simulink library "RABBIT_lib"  (R2015a)
settings: Solver=ode45  StartTime=0.0  StopTime=10.0  RelTol=1e-3
undefined symbols (not defined in the file or in its folder): dt, RABBITparams
undefined symbols (not defined in the file): RABBITsignals
settings Model: Creator=ffelici  LastModifiedBy=ffelici
settings SFSimCC: SimParseCustomCode=off

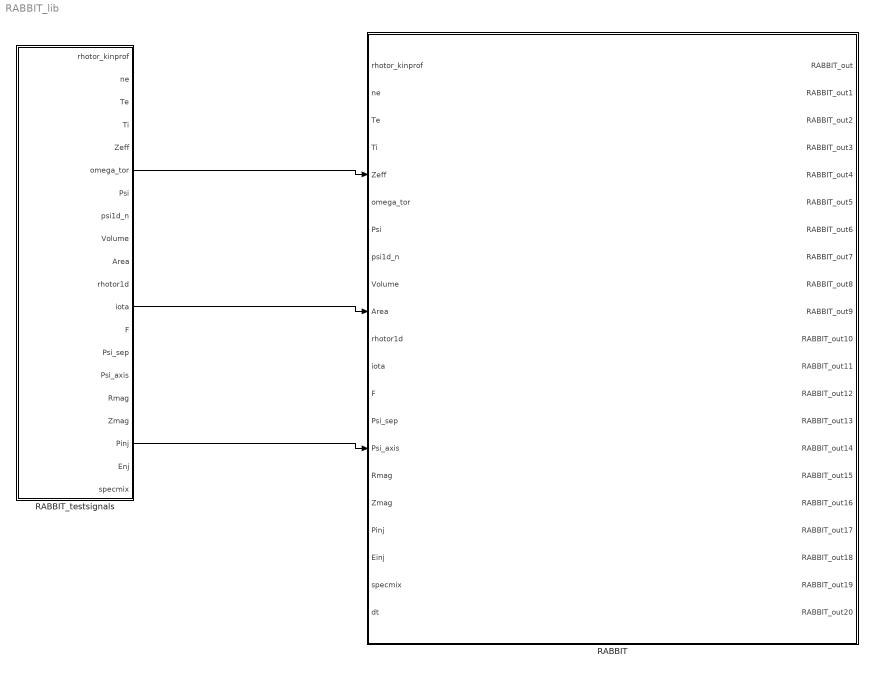
== system RABBIT_lib ==
  RABBIT : Subsystem  mask{RABBITparams=RABBITparams}
      mask prompts: RABBITparams "RABBIT parameters"
      mask Display:
      | image('rabbit.jpg')
      | 
      | port_label('input',1,'rhotorN kin profiles')
      | port_label('input',2,'ne [m^-3]')
      | port_label('input',3,'Te [eV]')
      | port_label('input',4,'Ti [eV]')
      | port_label('input',5,'Zeff')
      | port_label('input',6,'omega tor [rad/s]')
      | port_label('input',7,'Psi 2D [Wb/rad]')
      | port_label('input',8,'Psi1D grid [0-1]')
      | port_label('input',9,'Volume m^3')
      | port_label('input',10,'Area m^2')
      | port_label('input',11,'rhotorN eq profiles')
      | port_label('input',12,'iota = 1/q')
      | port_label('input',13,'F [Tm]')
      | port_label('input',14,'Psi_sep [Wb/rad]')
      | port_label('input',15,'Psi_axis [Wb/rad]')
      | port_label('input',16,'Rmag [m]')
      | port_label('input',17,'Zmag [m]')
      | port_label('input',18,'Pinj [W]')
      | port_label('input',19,'Einj [W]')
      | port_label('input',20,'specmix [-]')
      | port_label('input',21,'dt [s]')
      | 
      | 
      | port_label('output',1,'Power e- [W/m^3]')
      | port_label('output',2,'Power i+ [W/m^3]')
      | port_label('output',3,'Fast ion pressure [Pa]')
      | port_label('output',4,'Particle source [1/m^3/s]')
      | port_label('output',5,'Fast ion density [1/m^3]')
      | port_label('output',6,'Fast ion current density [A/m^2]')
      | port_label('output',7,'NB driven current [A/m^2]')
      | port_label('output',8,'Torque to electrons [Nm/m^3]')
      | port_label('output',9,'Torque to ions [Nm/m^3]')
      | port_label('output',10,'Torque to impurities [Nm/m^3]')
      | port_label('output',11,'Neutron rate [#/s/m^3]')
      | port_label('output',12,'rhotor out [-]')
      | port_label('output',13,'P e- total [W]')
      | port_label('output',14,'P i- total [W]')
      | port_label('output',15,'P shinethrough [W]')
      | port_label('output',16,'P rotation [W]')
      | port_label('output',17,'P orbit loss [W]')
      | port_label('output',18,'P CX loss [W]')
      | port_label('output',19,'Inb total [A]')
      | port_label('output',20,'exitflag')
      | port_label('output',21,'execution time [ms]')
  RABBIT_testsignals : Subsystem  mask{RABBITsignals=RABBITsignals, dt=dt}
      mask prompts: RABBITsignals "RABBITsignals structure"; dt "sample time"
  wires:
  RABBIT_testsignals/6(omega_tor) -> RABBIT/5(Zeff)
  RABBIT_testsignals/12(iota) -> RABBIT/10(Area)
  RABBIT_testsignals/18(Pinj) -> RABBIT/15(Psi_axis)

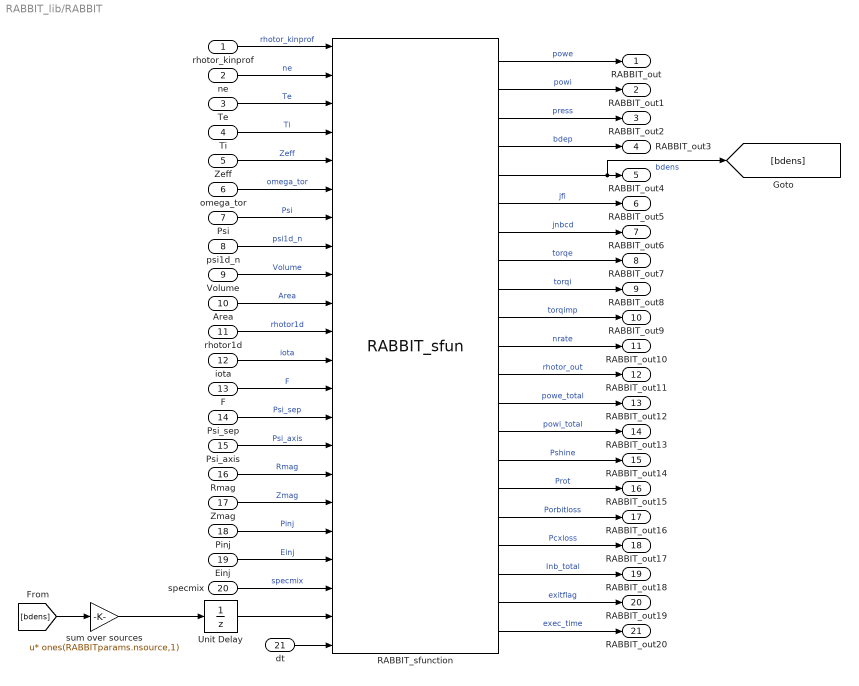
== system RABBIT_lib/RABBIT ==
  rhotor_kinprof : Inport  OutDataTypeStr=double  Interpolate=off
  ne : Inport  Port=2  OutDataTypeStr=double  Interpolate=off
  Te : Inport  Port=3  OutDataTypeStr=double  Interpolate=off
  Ti : Inport  Port=4  OutDataTypeStr=double  Interpolate=off
  Zeff : Inport  Port=5  OutDataTypeStr=double  Interpolate=off
  omega_tor : Inport  Port=6  OutDataTypeStr=double  Interpolate=off
  Psi : Inport  Port=7  OutDataTypeStr=double  Interpolate=off
  psi1d_n : Inport  Port=8  OutDataTypeStr=double  Interpolate=off
  Volume : Inport  Port=9  OutDataTypeStr=double  Interpolate=off
  Area : Inport  Port=10  OutDataTypeStr=double  Interpolate=off
  rhotor1d : Inport  Port=11  OutDataTypeStr=double  Interpolate=off
  iota : Inport  Port=12  OutDataTypeStr=double  Interpolate=off
  F : Inport  Port=13  OutDataTypeStr=double  Interpolate=off
  Psi_sep : Inport  Port=14  OutDataTypeStr=double  Interpolate=off
  Psi_axis : Inport  Port=15  OutDataTypeStr=double  Interpolate=off
  Rmag : Inport  Port=16  OutDataTypeStr=double  Interpolate=off
  Zmag : Inport  Port=17  OutDataTypeStr=double  Interpolate=off
  Pinj : Inport  Port=18  OutDataTypeStr=double  Interpolate=off
  Einj : Inport  Port=19  OutDataTypeStr=double  Interpolate=off
  specmix : Inport  Port=20  OutDataTypeStr=double  Interpolate=off
  dt : Inport  Port=21  OutDataTypeStr=double  PortDimensions=1  Interpolate=off
  RABBIT_sfunction : S-Function  FunctionName=RABBIT_sfun  Parameters=p.nsource,p.aplasma,p.zplasma,p.aimp,p.zimp,p.abeam,p.zbeam,p.xstart,p.xvec,p.beamwidthpoly,p.nv,p.nrhotor_out,p.R,p.Z,p.l,p.p  mask{p=RABBITparams}
      mask prompts: p "RABBITparams structure"
  Unit Delay : UnitDelay  SampleTime=-1
  sum over sources : Gain  Gain=ones(RABBITparams.nsource,1)  Multiplication=Matrix(u*K)
  RABBIT_out : Outport  OutDataTypeStr=double
  RABBIT_out1 : Outport  Port=2  OutDataTypeStr=double
  RABBIT_out2 : Outport  Port=3  OutDataTypeStr=double
  RABBIT_out3 : Outport  Port=4  OutDataTypeStr=double
  RABBIT_out4 : Outport  Port=5  OutDataTypeStr=double
  RABBIT_out5 : Outport  Port=6  OutDataTypeStr=double
  RABBIT_out6 : Outport  Port=7  OutDataTypeStr=double
  RABBIT_out7 : Outport  Port=8  OutDataTypeStr=double
  RABBIT_out8 : Outport  Port=9  OutDataTypeStr=double
  RABBIT_out9 : Outport  Port=10  OutDataTypeStr=double
  RABBIT_out10 : Outport  Port=11  OutDataTypeStr=double
  RABBIT_out11 : Outport  Port=12  OutDataTypeStr=double
  RABBIT_out12 : Outport  Port=13  OutDataTypeStr=double
  RABBIT_out13 : Outport  Port=14  OutDataTypeStr=double
  RABBIT_out14 : Outport  Port=15  OutDataTypeStr=double
  RABBIT_out15 : Outport  Port=16  OutDataTypeStr=double
  RABBIT_out16 : Outport  Port=17  OutDataTypeStr=double
  RABBIT_out17 : Outport  Port=18  OutDataTypeStr=double
  RABBIT_out18 : Outport  Port=19  OutDataTypeStr=double
  RABBIT_out19 : Outport  Port=20  OutDataTypeStr=double
  RABBIT_out20 : Outport  Port=21  OutDataTypeStr=double
  wires:
  Rmag/1 -> RABBIT_sfunction/16  "Rmag"
  RABBIT_sfunction/20 -> RABBIT_out19/1  "exitflag"
  sum over sources/1 -> Unit Delay/1
  dt/1 -> RABBIT_sfunction/22
  Zeff/1 -> RABBIT_sfunction/5  "Zeff"
  psi1d_n/1 -> RABBIT_sfunction/8  "psi1d_n"
  rhotor_kinprof/1 -> RABBIT_sfunction/1  "rhotor_kinprof"
  Te/1 -> RABBIT_sfunction/3  "Te"
  RABBIT_sfunction/14 -> RABBIT_out13/1  "powi_total"
  RABBIT_sfunction/15 -> RABBIT_out14/1  "Pshine"
  RABBIT_sfunction/16 -> RABBIT_out15/1  "Prot"
  RABBIT_sfunction/7 -> RABBIT_out6/1  "jnbcd"
  RABBIT_sfunction/8 -> RABBIT_out7/1  "torqe"
  RABBIT_sfunction/12 -> RABBIT_out11/1  "rhotor_out"
  RABBIT_sfunction/3 -> RABBIT_out2/1  "press"
  RABBIT_sfunction/6 -> RABBIT_out5/1  "jfi"
  RABBIT_sfunction/5 -> [bdens], RABBIT_out4/1  "bdens"
  RABBIT_sfunction/4 -> RABBIT_out3/1  "bdep"
  RABBIT_sfunction/2 -> RABBIT_out1/1  "powi"
  RABBIT_sfunction/1 -> RABBIT_out/1  "powe"
  [bdens] -> sum over sources/1
  Psi_sep/1 -> RABBIT_sfunction/14  "Psi_sep"
  Volume/1 -> RABBIT_sfunction/9  "Volume"
  specmix/1 -> RABBIT_sfunction/20  "specmix"
  Psi/1 -> RABBIT_sfunction/7  "Psi"
  rhotor1d/1 -> RABBIT_sfunction/11  "rhotor1d"
  Einj/1 -> RABBIT_sfunction/19  "Einj"
  Unit Delay/1 -> RABBIT_sfunction/21
  omega_tor/1 -> RABBIT_sfunction/6  "omega_tor"
  ne/1 -> RABBIT_sfunction/2  "ne"
  Ti/1 -> RABBIT_sfunction/4  "Ti"
  Area/1 -> RABBIT_sfunction/10  "Area"
  Psi_axis/1 -> RABBIT_sfunction/15  "Psi_axis"
  RABBIT_sfunction/21 -> RABBIT_out20/1  "exec_time"
  RABBIT_sfunction/19 -> RABBIT_out18/1  "Inb_total"
  RABBIT_sfunction/18 -> RABBIT_out17/1  "Pcxloss"
  RABBIT_sfunction/13 -> RABBIT_out12/1  "powe_total"
  RABBIT_sfunction/17 -> RABBIT_out16/1  "Porbitloss"
  Pinj/1 -> RABBIT_sfunction/18  "Pinj"
  iota/1 -> RABBIT_sfunction/12  "iota"
  F/1 -> RABBIT_sfunction/13  "F"
  RABBIT_sfunction/10 -> RABBIT_out9/1  "torqimp"
  RABBIT_sfunction/9 -> RABBIT_out8/1  "torqi"
  RABBIT_sfunction/11 -> RABBIT_out10/1  "nrate"
  Zmag/1 -> RABBIT_sfunction/17  "Zmag"

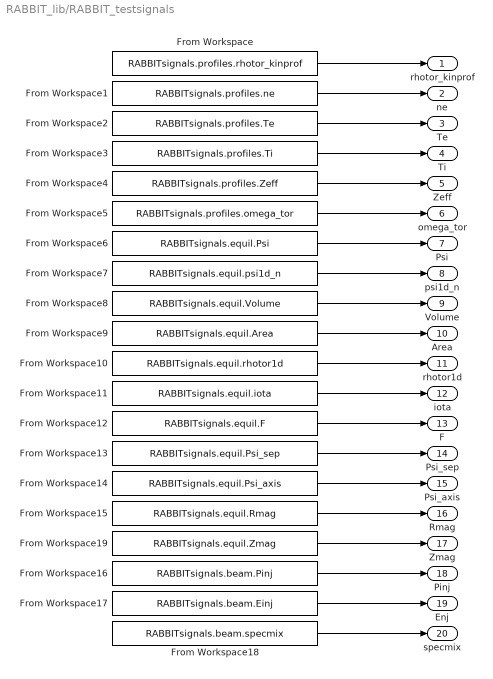
== system RABBIT_lib/RABBIT_testsignals ==
  From Workspace : FromWorkspace  VariableName=RABBITsignals.profiles.rhotor_kinprof  SampleTime=dt  OutputAfterFinalValue=Holding final value
  From Workspace1 : FromWorkspace  VariableName=RABBITsignals.profiles.ne  SampleTime=dt  OutputAfterFinalValue=Holding final value
  From Workspace10 : FromWorkspace  VariableName=RABBITsignals.equil.rhotor1d  SampleTime=dt  OutputAfterFinalValue=Holding final value
  From Workspace11 : FromWorkspace  VariableName=RABBITsignals.equil.iota  SampleTime=dt  OutputAfterFinalValue=Holding final value
  From Workspace12 : FromWorkspace  VariableName=RABBITsignals.equil.F  SampleTime=dt  OutputAfterFinalValue=Holding final value
  From Workspace13 : FromWorkspace  VariableName=RABBITsignals.equil.Psi_sep  SampleTime=dt  OutputAfterFinalValue=Holding final value
  From Workspace14 : FromWorkspace  VariableName=RABBITsignals.equil.Psi_axis  SampleTime=dt  OutputAfterFinalValue=Holding final value
  From Workspace15 : FromWorkspace  VariableName=RABBITsignals.equil.Rmag  SampleTime=dt  OutputAfterFinalValue=Holding final value
  From Workspace16 : FromWorkspace  VariableName=RABBITsignals.beam.Pinj  SampleTime=dt  OutputAfterFinalValue=Holding final value
  From Workspace17 : FromWorkspace  VariableName=RABBITsignals.beam.Einj  SampleTime=dt  OutputAfterFinalValue=Holding final value
  From Workspace18 : FromWorkspace  VariableName=RABBITsignals.beam.specmix  SampleTime=dt  OutputAfterFinalValue=Holding final value
  From Workspace19 : FromWorkspace  VariableName=RABBITsignals.equil.Zmag  SampleTime=dt  OutputAfterFinalValue=Holding final value
  From Workspace2 : FromWorkspace  VariableName=RABBITsignals.profiles.Te  SampleTime=dt  OutputAfterFinalValue=Holding final value
  From Workspace3 : FromWorkspace  VariableName=RABBITsignals.profiles.Ti  SampleTime=dt  OutputAfterFinalValue=Holding final value
  From Workspace4 : FromWorkspace  VariableName=RABBITsignals.profiles.Zeff  SampleTime=dt  OutputAfterFinalValue=Holding final value
  From Workspace5 : FromWorkspace  VariableName=RABBITsignals.profiles.omega_tor  SampleTime=dt  OutputAfterFinalValue=Holding final value
  From Workspace6 : FromWorkspace  VariableName=RABBITsignals.equil.Psi  SampleTime=dt  OutputAfterFinalValue=Holding final value
  From Workspace7 : FromWorkspace  VariableName=RABBITsignals.equil.psi1d_n  SampleTime=dt  OutputAfterFinalValue=Holding final value
  From Workspace8 : FromWorkspace  VariableName=RABBITsignals.equil.Volume  SampleTime=dt  OutputAfterFinalValue=Holding final value
  From Workspace9 : FromWorkspace  VariableName=RABBITsignals.equil.Area  SampleTime=dt  OutputAfterFinalValue=Holding final value
  "  rhotor_kinprof" : Outport
  ne : Outport  Port=2
  Te : Outport  Port=3
  Ti : Outport  Port=4
  Zeff : Outport  Port=5
  omega_tor : Outport  Port=6
  Psi : Outport  Port=7
  psi1d_n : Outport  Port=8
  Volume : Outport  Port=9
  Area : Outport  Port=10
  rhotor1d : Outport  Port=11
  iota : Outport  Port=12
  F : Outport  Port=13
  Psi_sep : Outport  Port=14
  Psi_axis : Outport  Port=15
  Rmag : Outport  Port=16
  Zmag : Outport  Port=17
  Pinj : Outport  Port=18
  Enj : Outport  Port=19
  specmix : Outport  Port=20
  wires:
  From Workspace10/1 -> rhotor1d/1
  From Workspace15/1 -> Rmag/1
  From Workspace13/1 -> Psi_sep/1
  From Workspace11/1 -> iota/1
  From Workspace8/1 -> Volume/1
  From Workspace19/1 -> Zmag/1
  From Workspace9/1 -> Area/1
  From Workspace/1 -> "  rhotor_kinprof"/1
  From Workspace7/1 -> psi1d_n/1
  From Workspace18/1 -> specmix/1
  From Workspace14/1 -> Psi_axis/1
  From Workspace12/1 -> F/1
  From Workspace1/1 -> ne/1
  From Workspace16/1 -> Pinj/1
  From Workspace5/1 -> omega_tor/1
  From Workspace17/1 -> Enj/1
  From Workspace3/1 -> Ti/1
  From Workspace4/1 -> Zeff/1
  From Workspace2/1 -> Te/1
  From Workspace6/1 -> Psi/1
